simulink model "chapter6_motor_simulation_simulink"  (R2022b)
settings: Solver=ode4  StartTime=0.0  StopTime=10.0  FixedStep=0.001  RelTol=1e-3
values from neighbouring files (symbols this model uses):
  Ke = 1    [chapter6_motor_simulation.m]
  Ks = 0.1    [chapter6_motor_simulation.m]
  Kt = 1    [chapter6_motor_simulation.m]
  R = 0.1    [chapter6_motor_simulation.m]
  Tau_m = R*(J+Ks^2*Js)/(Kt*Ke)    (= 1.001)    [chapter6_motor_simulation.m]
settings Model: Creator=craft  LastModifiedBy=craft

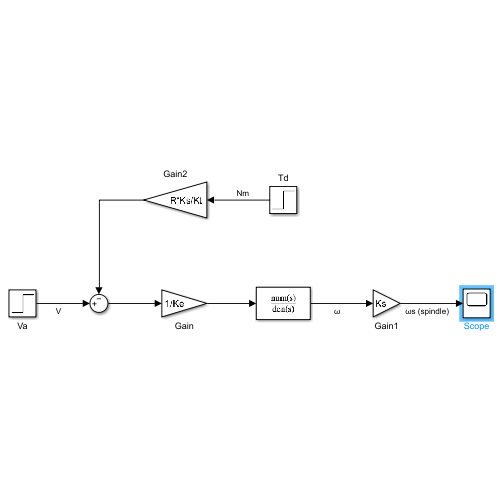
[thumbnail: Simulink's stored preview of the top-level diagram]
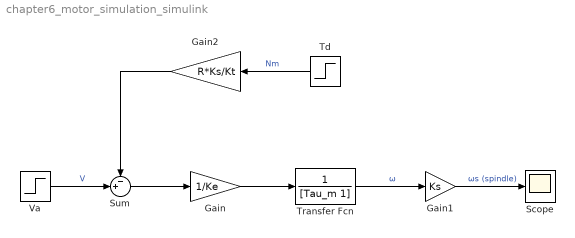
== system chapter6_motor_simulation_simulink ==
  Gain : Gain  Gain=1/Ke
  Gain1 : Gain  Gain=Ks
  Gain2 : Gain  Gain=R*Ks/Kt
  Scope : Scope
  Sum : Sum  Inputs=-+|
  Td : Step  After=0  SampleTime=0
  Transfer Fcn : TransferFcn  Denominator=[Tau_m 1]
  Va : Step  SampleTime=0
  wires:
  Td/1 -> Gain2/1  "Nm"
  Gain2/1 -> Sum/1
  Va/1 -> Sum/2  "V"
  Sum/1 -> Gain/1
  Transfer Fcn/1 -> Gain1/1  "ω"
  Gain1/1 -> Scope/1  "ωs (spindle)"
  Gain/1 -> Transfer Fcn/1
